simulink model "Current_PI"  (R2020a)
settings: Solver=VariableStepAuto  StartTime=0.0  StopTime=0.2  RelTol=1e-3
values from neighbouring files (symbols this model uses):
  Ki_c = Kp_c * wc_c    (= 40)    [parameter.m]
  Kp_c = Gain_c * 1/50    (= 2)    [parameter.m]
settings Model: Creator=ykamatan  LastModifiedBy=ykamatan
settings SolverCC: ZeroCrossAlgorithm=Adaptive
settings DataIOCC: SaveOutput=off  SaveTime=off
settings DebuggingCC: IgnoredZcDiagnostic=none

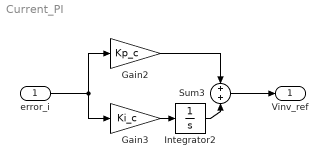
== system Current_PI ==
  error_i : Inport  OutDataTypeStr=double  PortDimensions=1  SampleTime=0
  Gain2 : Gain  Gain=Kp_c
  Gain3 : Gain  Gain=Ki_c
  Integrator2 : Integrator
  Sum3 : Sum  Inputs=+|+
  Vinv_ref : Outport  OutDataTypeStr=double  PortDimensions=1  SampleTime=0
  wires:
  error_i/1 -> Gain3/1, Gain2/1
  Integrator2/1 -> Sum3/2
  Gain2/1 -> Sum3/1
  Gain3/1 -> Integrator2/1
  Sum3/1 -> Vinv_ref/1
